simulink model "WiperControl_Automation"  (R2020b)
settings: Solver=FixedStepAuto  StartTime=0.0  StopTime=10  MaxStep=0.01  RelTol=1e-3
undefined symbols (not defined in the file or in its folder): sigbuilder_block
settings Model: Creator=99003778  LastModifiedBy=99003778
settings DataIOCC: SaveState=on  LoggingToFile=on
settings DebuggingCC: ArithmeticOperatorsInVariantConditions=warning
settings SFSimCC: CustomCodeUndefinedFunction=UseInterfaceOnly

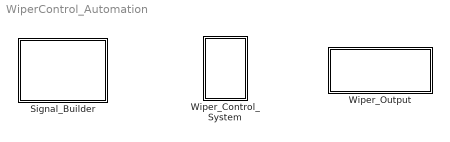
== system WiperControl_Automation ==
  Signal_Builder : Subsystem
  Wiper_Control_System : Subsystem
  Wiper_Output : Subsystem

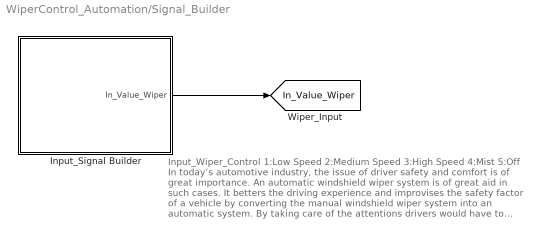
== system WiperControl_Automation/Signal_Builder ==
  note: Input_Wiper_Control
      | 1:Low Speed
      | 2:Medium Speed
      | 3:High Speed
      | 4:Mist
      | 5:Off
      | In today’s automotive industry, the issue of driver safety and comfort is of great importance. An automatic windshield wiper system is of great aid in such cases. It betters the driving experience and improvises the safety factor of a vehicle by converting the manual windshield wiper system into an automatic system. By taking care of the attentions drivers would have to devote to control a manual system, an automatic wiper system helps them to concentrate more on driving safely. Although, few automated windshield wiper systems are available in the automotive market, they are very costly and not very effective.
  Input_Signal Builder : Subsystem  Tag=STV Subsys  LoadFcn=sigbuilder_block('load',[339 188.25 550.5 359.25 ]);  StartFcn=sigbuilder_block('start');  StopFcn=sigbuilder_block('stop');  ClipboardFcn=sigbuilder_block('clipboard');  mask(Sigbuilder block){tuvar=[0:10]}
      mask help: Simulink:masks:SigbuilderBlock_MD
      mask init:
      | if ~strcmp(get_param(bdroot(gcbh),'SimulationStatus'),'stopped') tuvar = sigbuilder_block('maskInit'); end
      settings: CopyFcn=sigbuilder_block('copy');  DeleteFcn=sigbuilder_block('delete');  ModelCloseFcn=sigbuilder_block('modelClose');  PreSaveFcn=sigbuilder_block('preSave');  PauseFcn=sigbuilder_block('pause');  ContinueFcn=sigbuilder_block('continue');  NameChangeFcn=sigbuilder_block('namechange');  OpenFcn=sigbuilder_block('open',[339 188.25 550.5 359.25 ]);  CloseFcn=sigbuilder_block('close');
      mask Display: plot(0, 0, 100, 100,[2, 2, 32, 32, 2], [68, 8, 8, 68, 68],[32, 2], [38, 38], [32, 19, 2],[53, 60, 44], [32, 17, 17, 2],[16, 16, 31, 31]);txt = getActiveGroup(gcbh);text(2, 100, txt,'verticalAlignment', 'top');
  tag scope: In_Value_Wiper=global
  wires:
  Input_Signal Builder/1(In_Value_Wiper) -> [In_Value_Wiper]

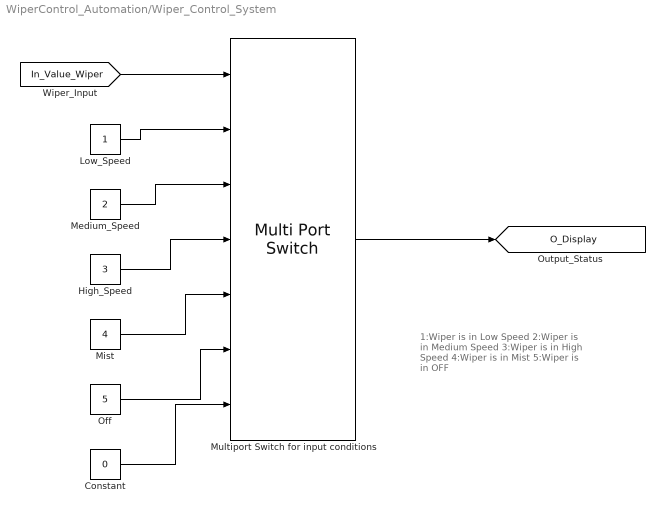
== system WiperControl_Automation/Wiper_Control_System ==
  note: 1:Wiper is in Low Speed
      | 2:Wiper is in Medium Speed
      | 3:Wiper is in High Speed
      | 4:Wiper is in Mist
      | 5:Wiper is in OFF
  Constant : Constant  Value=0
  High_Speed : Constant  Value=3
  Low_Speed : Constant
  Medium_Speed : Constant  Value=2
  Mist : Constant  Value=4
  Multiport Switch for input conditions : MultiPortSwitch  Inputs=6  DiagnosticForDefault=None
  Off : Constant  Value=5
  tag scope: O_Display=global
  wires:
  [In_Value_Wiper] -> Multiport Switch for input conditions/1
  Low_Speed/1 -> Multiport Switch for input conditions/2
  Mist/1 -> Multiport Switch for input conditions/5
  Medium_Speed/1 -> Multiport Switch for input conditions/3
  Multiport Switch for input conditions/1 -> [O_Display]
  High_Speed/1 -> Multiport Switch for input conditions/4
  Off/1 -> Multiport Switch for input conditions/6
  Constant/1 -> Multiport Switch for input conditions/7

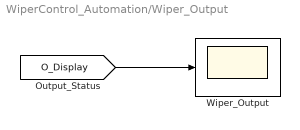
== system WiperControl_Automation/Wiper_Output ==
  Wiper_Output : Scope
  wires:
  [O_Display] -> Wiper_Output/1

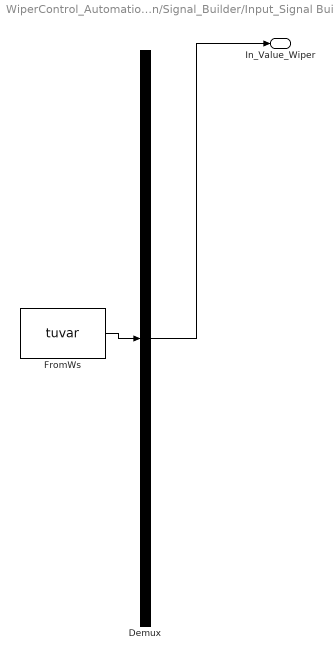
== system WiperControl_Automation/Signal_Builder/Input_Signal Builder ==
  Demux : Demux  Tag=STV Demux  Outputs=1
      settings: DisplayOption=none
  FromWs : FromWorkspace  Tag=STV FromWs  VariableName=tuvar
      SigBuilderData=|
      | common.afterFinalStr = 'Extrapolate'
      | common.sampleTime = 0
      | dataSet.timeRange = [0 25]
      | dataSet.name = 'Group 1'
      | sbobj.Groups.Name = 'Group 1'
      | sbobj.Groups.Signals.Name = 'In_Value_Wiper'
      | sbobj.Groups.Signals.XData = [0 1 2 3 4 5 6 7 8 9 10 11 12 13 14 15 16 17 18 19 20 21 22 23 24 25]
      | sbobj.Groups.Signals.YData = [1 2 3 4 5 1 2 3 4 5 1 2 3 4 5 1 2 3 4 5 1 2 3 4 5 2]
      | sbobj.Groups.TimeRange = [0 25]
  In_Value_Wiper : Outport  Tag=STV Outport
  wires:
  FromWs/1 -> Demux/1
  Demux/1 -> In_Value_Wiper/1
